simulink model "DFNN_EFS"  (R2022a)
settings: Solver=ode1  StartTime=0.0  StopTime=5  FixedStep=0.001  RelTol=1e-3
libraries: roblocks x1
settings Model: Creator=DELL  LastModifiedBy=qinyi
settings DebuggingCC: UnconnectedInputMsg=warning  UnconnectedOutputMsg=warning  UnconnectedLineMsg=warning
settings RTWCC: DLArmComputeVersion=19.05

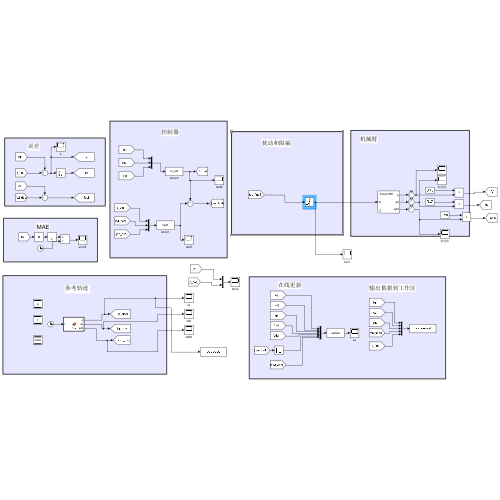
[thumbnail: Simulink's stored preview of the top-level diagram]
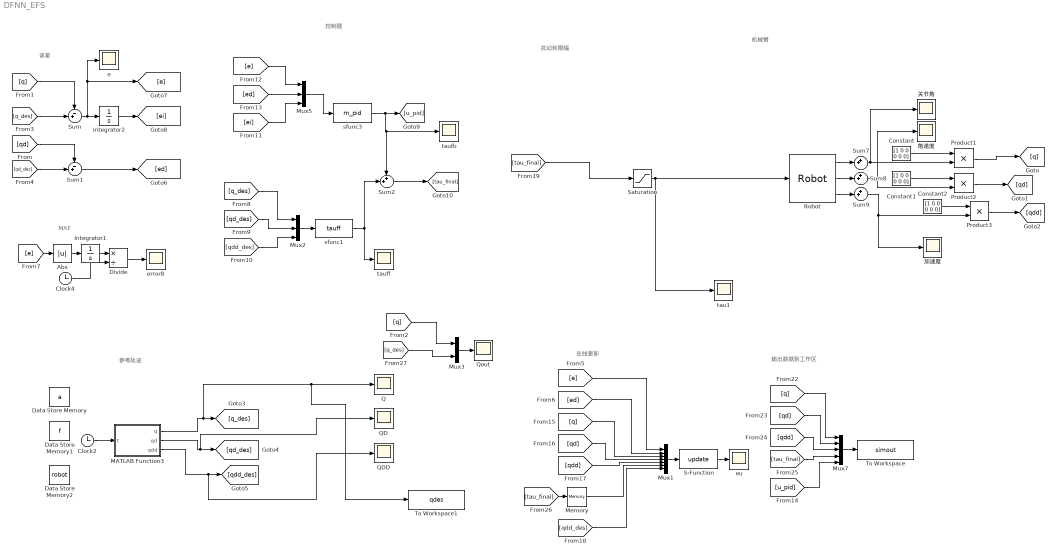
== system DFNN_EFS ==
  note: 在线更新
  note: MAE
  note: 机械臂
  note: 扰动和限幅
  note: 控制器
  note: 误差
  note: 参考轨迹
  note: 输出数据到工作区
  Abs : Abs  SaturateOnIntegerOverflow=off
  Clock2 : Clock
  Clock4 : Clock
  Constant : Constant  Value=[1 0 0 0 0 0]
  Constant1 : Constant  Value=[1 0 0 0 0 0]
  Constant2 : Constant  Value=[1 0 0 0 0 0]
  Data Store Memory : DataStoreMemory  DataStoreName=a  ReadBeforeWriteMsg=warning  WriteAfterWriteMsg=warning  WriteAfterReadMsg=warning  InitialValue=rand(10,6)  ShowAdditionalParam=off  OutDataTypeStr=double
  Data Store Memory1 : DataStoreMemory  DataStoreName=f  ReadBeforeWriteMsg=warning  WriteAfterWriteMsg=warning  WriteAfterReadMsg=warning  InitialValue=rand(10,6)  ShowAdditionalParam=off  OutDataTypeStr=double
  Data Store Memory2 : DataStoreMemory  DataStoreName=robot  ReadBeforeWriteMsg=warning  WriteAfterWriteMsg=warning  WriteAfterReadMsg=warning  InitialValue=rand(10,6)  ShowAdditionalParam=off  OutDataTypeStr=double
  Divide : Product  Inputs=*/
  Integrator1 : Integrator
  Integrator2 : Integrator  LimitOutput=on  UpperSaturationLimit=0.01  LowerSaturationLimit=-0.01
  MATLAB Function3 : MATLAB Function  TreatAsAtomicUnit=on
  Memory : Memory
  Mux1 : Mux  Inputs=7
  Mux2 : Mux  Inputs=3
  Mux3 : Mux  Inputs=2
  Mux5 : Mux  Inputs=3
  Mux7 : Mux  Inputs=5
  Product1 : Product
  Product2 : Product
  Product3 : Product
  Q : Scope
  QD : Scope
  QDD : Scope
  Qout : Scope
  Robot : roblocks/Arm/Robot  robot=p560  q0=[90 0 30 30 0 0]*pi/180
      link override Integrator: InitialCondition=0
      link override Integrator1: InitialCondition=[0 90 -90 30 0 0]'*pi/180
      link override S-Function: Parameters=p560
  S-Function : S-Function  FunctionName=update  SFunctionDeploymentMode=off  EnableBusSupport=off
  Saturation : Saturate  UpperLimit=2000  LowerLimit=-2000
  Sum : Sum  Inputs=-+|
  Sum1 : Sum  Inputs=-+|
  Sum{2,7..9} (4 alike) : Sum  Inputs=++|
  To Workspace : ToWorkspace  VariableName=simout  SaveFormat=Timeseries  SampleTime=-1
  To Workspace1 : ToWorkspace  VariableName=qdes  SaveFormat=Timeseries  SampleTime=-1
  e : Scope
  error8 : Scope
  eu : Scope
  sfunc1 : S-Function  FunctionName=tauff  Parameters=p560  SFunctionDeploymentMode=off  EnableBusSupport=off
  sfunc3 : S-Function  FunctionName=m_pid  SFunctionDeploymentMode=off  EnableBusSupport=off
  tau1 : Scope
  taufb : Scope
  tauff : Scope
  关节角 : Scope
  加速度 : Scope
  角速度 : Scope
  wires:
  Sum/1 -> Integrator2/1, e/1, [e]
  Sum1/1 -> [ed]
  Mux2/1 -> sfunc1/1
  Abs/1 -> Integrator1/1
  Integrator1/1 -> Divide/1
  Divide/1 -> error8/1
  Mux5/1 -> sfunc3/1
  S-Function/1 -> eu/1
  Mux7/1 -> To Workspace/1
  sfunc1/1 -> Sum2/2, tauff/1
  Mux1/1 -> S-Function/1
  Sum7/1 -> Product1/2, 关节角/1
  Sum8/1 -> 角速度/1, Product2/2
  Sum9/1 -> Product3/2, 加速度/1
  Integrator2/1 -> [ei]
  Clock2/1 -> MATLAB Function3/1(t)
  MATLAB Function3/1(q) -> To Workspace1/1, Q/1, [q_des]
  MATLAB Function3/2(qd) -> QD/1, [qd_des]
  MATLAB Function3/3(qdd) -> QDD/1, [qdd_des]
  Clock4/1 -> Divide/2
  [q] -> Sum/1
  [qd] -> Sum1/1
  [q_des] -> Sum/2
  [qd_des] -> Sum1/2
  [e] -> Mux1/1
  [ed] -> Mux1/2
  [e] -> Abs/1
  [q_des] -> Mux2/1
  [qd_des] -> Mux2/2
  [qdd_des] -> Mux2/3
  [e] -> Mux5/1
  [ed] -> Mux5/2
  [ei] -> Mux5/3
  sfunc3/1 -> taufb/1, Sum2/1, [u_pid]
  [u_pid] -> Mux7/5
  [q] -> Mux1/3
  [qd] -> Mux1/4
  [qdd] -> Mux1/5
  [qdd_des] -> Mux1/7
  Sum2/1 -> [tau_final]
  Robot/1 -> Sum7/2
  Robot/2 -> Sum8/2
  Robot/3 -> Sum9/2
  [q] -> Mux7/1
  [qd] -> Mux7/2
  [qdd] -> Mux7/3
  [tau_final] -> Mux7/4
  [tau_final] -> Memory/1
  [tau_final] -> Saturation/1
  Saturation/1 -> Robot/1, tau1/1
  Constant/1 -> Product1/1
  Product2/1 -> [qd]
  Product3/1 -> [qdd]
  Constant1/1 -> Product2/1
  Constant2/1 -> Product3/1
  Product1/1 -> [q]
  Mux3/1 -> Qout/1
  [q] -> Mux3/1
  [q_des] -> Mux3/2
  Memory/1 -> Mux1/6

== matlab function DFNN_EFS/MATLAB Function3 ==
  settings: updateMethod=DISCRETE
  data: t input; q output; qd output; qdd output; a data_store_memory; f data_store_memory
function [q,qd,qdd] = fcn(t)
if(t >= 2.5)
    B=[80 70 70 0 0 0]*pi/180;
    q = [0 0 0 0 0 0]'+[0 90 -90 0 0 0]'*pi/180;
    qd = zeros(6,1);
    qdd = zeros(6,1);
else
    B=[80 70 70 0 0 0]*pi/180;
    q = [0.5 0.5 0.5 0.5 0.5 0.5]'+[0 90 -90 0 0 0]'*pi/180;
    qd = zeros(6,1);
    qdd = zeros(6,1);
end
